simulink subsystem "data_logging_for_ego_veh_subsystem"  (R2025a)
settings: Solver=VariableStepAuto  StartTime=0.0  StopTime=10.0  RelTol=1e-3
settings Model: Creator=admin  LastModifiedBy=admin

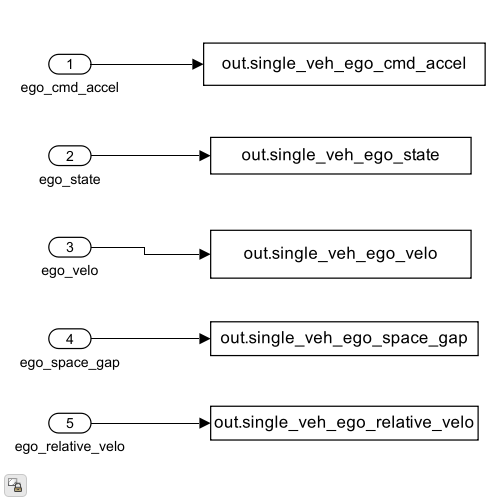
[thumbnail: Simulink's stored preview of the top-level diagram]
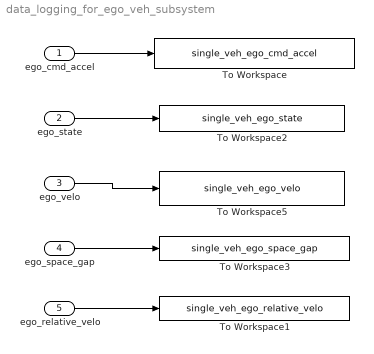
== system data_logging_for_ego_veh_subsystem ==
  ego_cmd_accel : Inport
  ego_state : Inport  Port=2
  ego_velo : Inport  Port=3
  ego_space_gap : Inport  Port=4
  ego_relative_velo : Inport  Port=5
  To Workspace : ToWorkspace  VariableName=single_veh_ego_cmd_accel  SaveFormat=Structure With Time  SampleTime=-1
  To Workspace1 : ToWorkspace  VariableName=single_veh_ego_relative_velo  SaveFormat=Structure With Time  SampleTime=-1
  To Workspace2 : ToWorkspace  VariableName=single_veh_ego_state  SaveFormat=Structure With Time  SampleTime=-1
  To Workspace3 : ToWorkspace  VariableName=single_veh_ego_space_gap  SaveFormat=Structure With Time  SampleTime=-1
  To Workspace5 : ToWorkspace  VariableName=single_veh_ego_velo  SaveFormat=Structure With Time  SampleTime=-1
  wires:
  ego_state/1 -> To Workspace2/1
  ego_space_gap/1 -> To Workspace3/1
  ego_cmd_accel/1 -> To Workspace/1
  ego_velo/1 -> To Workspace5/1
  ego_relative_velo/1 -> To Workspace1/1
